simulink model "fig423"  (Simulink 3.00)
settings: Solver=ode45  SolverMode=SingleTasking  StartTime=0.0  StopTime=10.0  RelTol=1e-3  AbsTol=1e-6
undefined symbols (not defined in the file or in its folder): ka

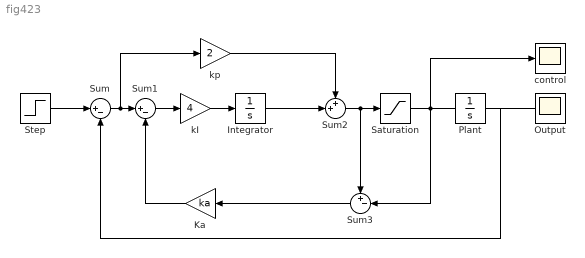
== system fig423 ==
  Integrator : Integrator  ExternalReset=none  InitialConditionSource=internal  InitialCondition=0  LimitOutput=off  UpperSaturationLimit=inf  LowerSaturationLimit=-inf  ShowSaturationPort=off  ShowStatePort=off  AbsoluteTolerance=auto
  Ka : Gain  Orientation=left  Gain=ka  SaturateOnIntegerOverflow=on
  Output : Scope
      settings: TickLabels=on  TimeRange=auto  YMin=-5  YMax=5  SaveName=yantib  DataFormat=Matrix
  Plant : Integrator  ExternalReset=none  InitialConditionSource=internal  InitialCondition=0  LimitOutput=off  UpperSaturationLimit=inf  LowerSaturationLimit=-inf  ShowSaturationPort=off  ShowStatePort=off  AbsoluteTolerance=auto
  Saturation : Saturate  UpperLimit=1.0  LowerLimit=-1.0
  Step : Step  Time=.2  Before=0  After=1  SampleTime=0.01
  Sum : Sum  Inputs=|+-  SaturateOnIntegerOverflow=on
  Sum1 : Sum  Inputs=|+-  SaturateOnIntegerOverflow=on
  Sum2 : Sum  Inputs=++|  SaturateOnIntegerOverflow=on
  Sum3 : Sum  Orientation=left  Inputs=+-|  SaturateOnIntegerOverflow=off
  control : Scope
      settings: TickLabels=on  TimeRange=auto  YMin=-5  YMax=5  SaveName=uantib  DataFormat=Matrix
  kI : Gain  Gain=4  SaturateOnIntegerOverflow=off
  kp : Gain  Gain=2  SaturateOnIntegerOverflow=off
  wires:
  kI/1 -> Integrator/1
  Plant/1 -> Output/1, Sum/2
  Saturation/1 -> Sum3/2, Plant/1, control/1
  Sum1/1 -> kI/1
  Sum3/1 -> Ka/1
  Step/1 -> Sum/1
  Ka/1 -> Sum1/2
  Sum2/1 -> Saturation/1, Sum3/1
  Integrator/1 -> Sum2/2
  kp/1 -> Sum2/1
  Sum/1 -> Sum1/1, kp/1
